simulink model "NewOrbitSimulation"  (R2015a)
settings: Solver=ode45  StartTime=0.0  StopTime=1000  FixedStep=.1  RelTol=1e-9
InitFcn:
  | PlanetSelect;
StopFcn:
  | TotalDeltaV
values from neighbouring files (symbols this model uses):
  Aero_On = 1    [PlanetSelect.m]
  AtmoData = 0    [PlanetSelect.m]
  Cd = 2    [PlanetSelect.m]
  Cl = 2    [PlanetSelect.m]
  Coasting_Parameter = 306.412    [PlanetSelect.m]
  Constant_Drag_On = 1    [PlanetSelect.m]
  Constant_Lift_On = 1    [PlanetSelect.m]
  CraftInitialP = [Px;Py]    [PlanetSelect.m]
  CraftInitialV = [Vx;Vy]    [PlanetSelect.m]
  Drag_On = 1    [PlanetSelect.m]
  g0 = 9.80665    [PlanetSelect.m]
  LastStage = size(ThrustMassData,1)    [PlanetSelect.m]
  Lift_On = 0    [PlanetSelect.m]
  PitchOverAlt = 1000    [PlanetSelect.m]
  PitchOverAngle = 7.5    [PlanetSelect.m]
  PitchSwitch = .5    (= 0.5)    [PlanetSelect.m]
  RefSurfArea = 10.8    [PlanetSelect.m]
  TargetOrbit = 100000-GndAlt_planet    [PlanetSelect.m]
  Throttle = 1.5*g0*ThrustMassData(1,1)/(1000*ThrustMassData(1,3))    [PlanetSelect.m]
  ThrustEnable = 1    [PlanetSelect.m]
undefined symbols (not defined in the file or in its folder): AtmoAlt_planet, DragData, GM_planet, GndAlt_planet, Omega_planet, R_planet
libraries: simulink_extras x6, dspmathops x5, simulink x3, vrlib x2
settings Model: PauseTimes=122  SnapshotInterval=1  Creator=raulm_000  LastModifiedBy=raulm_000
settings DataIOCC: ExternalInput=[Throttle,SSIGN]  LimitDataPoints=off  SaveFinalState=on

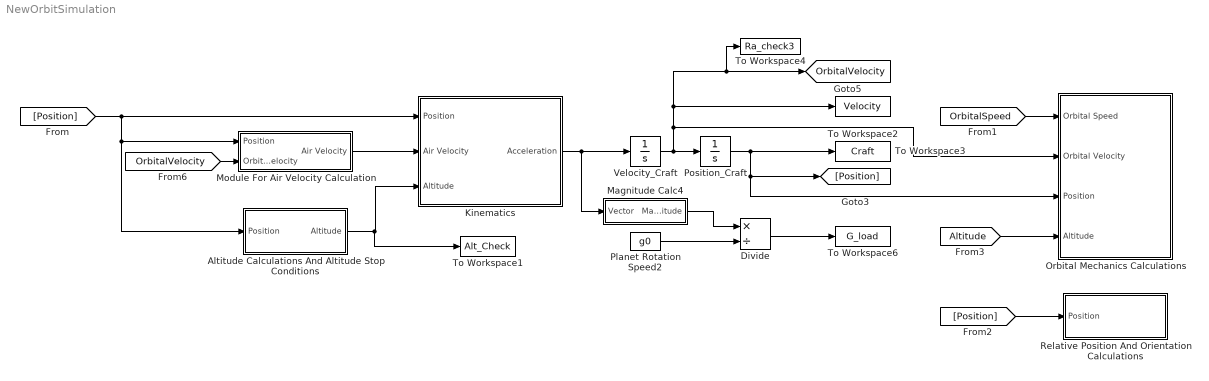
== system NewOrbitSimulation ==
  Altitude Calculations And Altitude Stop Conditions : Subsystem
  Divide : Product  Inputs=*/
  Kinematics : Subsystem
  Magnitude Calc4 : Subsystem
  Module For Air Velocity Calculation : Subsystem
  Orbital Mechanics Calculations : Subsystem
  Planet Rotation Speed2 : Constant  Value=g0
  Position_Craft : Integrator  InitialCondition=CraftInitialP
  Relative Position And Orientation Calculations : Subsystem
  To Workspace1 : ToWorkspace  VariableName=Alt_Check  SampleTime=-1
      settings: MaxDataPoints=1
  To Workspace2 : ToWorkspace  VariableName=Velocity  SampleTime=-1
  To Workspace3 : ToWorkspace  VariableName=Craft  SampleTime=-1
  To Workspace4 : ToWorkspace  VariableName=Ra_check3  SampleTime=-1
      settings: MaxDataPoints=1
  To Workspace6 : ToWorkspace  VariableName=G_load  SampleTime=-1
  Velocity_Craft : Integrator  InitialCondition=CraftInitialV-[.1;0]
  tag scope: OrbitalVelocity=global
  wires:
  Velocity_Craft/1 -> Position_Craft/1, To Workspace4/1, [OrbitalVelocity], To Workspace2/1, Orbital Mechanics Calculations/2(Orbital Velocity)
  Kinematics/1("Acceleration ") -> Velocity_Craft/1, Magnitude Calc4/1(Vector)
  Magnitude Calc4/1("Magnitude ") -> Divide/1
  Planet Rotation Speed2/1 -> Divide/2
  Divide/1 -> To Workspace6/1
  [OrbitalSpeed] -> Orbital Mechanics Calculations/1(Orbital Speed)
  [Altitude] -> Orbital Mechanics Calculations/4(Altitude)
  Position_Craft/1 -> Orbital Mechanics Calculations/3(Position), [Position], To Workspace3/1
  Module For Air Velocity Calculation/1(Air Velocity) -> Kinematics/2(Air Velocity)
  [Position] -> Module For Air Velocity Calculation/1(Position), Altitude Calculations And Altitude Stop Conditions/1(Position), Kinematics/1(Position)
  Altitude Calculations And Altitude Stop Conditions/1(Altitude) -> To Workspace1/1, Kinematics/3("Altitude ")
  [OrbitalVelocity] -> Module For Air Velocity Calculation/2(Orbital Velocity)
  [Position] -> Relative Position And Orientation Calculations/1(Position)

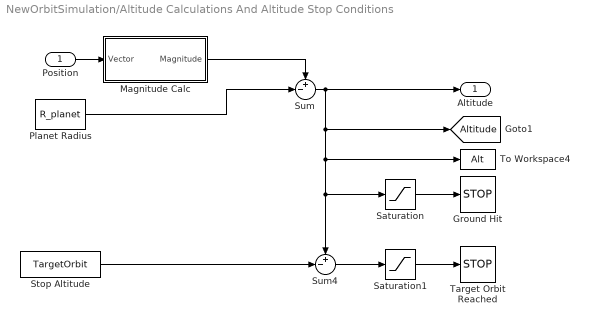
== system NewOrbitSimulation/Altitude Calculations And Altitude Stop Conditions ==
  Position : Inport
  " Target Orbit Reached" : Stop
  Ground Hit : Stop
  Magnitude Calc : Subsystem
  "Planet Radius " : Constant  Value=R_planet
  Saturation : Saturate  UpperLimit=0
  Saturation1 : Saturate  UpperLimit=1  LowerLimit=0
  Stop Altitude : Constant  Value=TargetOrbit
  Sum : Sum  Inputs=+-|
  Sum4 : Sum  Inputs=+-|
  To Workspace4 : ToWorkspace  VariableName=Alt  SampleTime=-1
  Altitude : Outport
  tag scope: Altitude=global
  wires:
  Magnitude Calc/1("Magnitude ") -> Sum/1
  "Planet Radius "/1 -> Sum/2
  Sum/1 -> Sum4/1, Saturation/1, To Workspace4/1, [Altitude], Altitude/1
  Saturation/1 -> Ground Hit/1
  Stop Altitude/1 -> Sum4/2
  Sum4/1 -> Saturation1/1
  Saturation1/1 -> " Target Orbit Reached"/1
  Position/1 -> Magnitude Calc/1(Vector)

== system NewOrbitSimulation/Kinematics ==
  Position : Inport
  Air Velocity : Inport  Port=2
  "Altitude " : Inport  Port=3
  Aerodynamics : Subsystem
  Gravitational Acceleration : Subsystem
  Sum3 : Sum  Inputs=+++
  Thrust : Subsystem
  "Acceleration " : Outport
  wires:
  Position/1 -> Thrust/2(Position), Gravitational Acceleration/1(Position)
  Air Velocity/1 -> Thrust/3(AirVelocity), Aerodynamics/1(Air Velocity)
  "Altitude "/1 -> Thrust/1(Altitude), Aerodynamics/2("Altitude ")
  Aerodynamics/1("Aeroaccel ") -> Sum3/2
  Gravitational Acceleration/1("Gavity ") -> Sum3/1
  Sum3/1 -> "Acceleration "/1
  Thrust/1("ThrustAccel ") -> Sum3/3

== system NewOrbitSimulation/Magnitude Calc4 ==
  Vector : Inport
  Add : Sum
  Demux : Demux  Outputs=2
  Math Function : Math  Operator=square  SaturateOnIntegerOverflow=on
  Math Function1 : Math  Operator=square  SaturateOnIntegerOverflow=on
  Sqrt : Sqrt  SaturateOnIntegerOverflow=on
  "Magnitude " : Outport
  wires:
  Demux/1 -> Math Function1/1
  Demux/2 -> Math Function/1
  Math Function/1 -> Add/2
  Add/1 -> Sqrt/1
  Vector/1 -> Demux/1
  Math Function1/1 -> Add/1
  Sqrt/1 -> "Magnitude "/1

== system NewOrbitSimulation/Module For Air Velocity Calculation ==
  Position : Inport
  Orbital Velocity : Inport  Port=2
  Cross Product1 : vrlib/Utilities/Cross Product
  Magnitude Calc1 : Subsystem
  Magnitude Calc3 : Subsystem
  Mux : Mux  Inputs=2
  Planet Rotation Speed1 : Constant  Value=0
  Sum2 : Sum  Inputs=|-+
  Air Velocity : Outport
  tag scope: OrbitalSpeed=global
  wires:
  [Planet_Ang_Vec] -> Cross Product1/1
  Cross Product1/1 -> Magnitude Calc3/1(3-in)
  Mux/1 -> Cross Product1/2
  Planet Rotation Speed1/1 -> Mux/2
  Magnitude Calc3/1("2-out ") -> Sum2/1
  Magnitude Calc1/1("Magnitude ") -> [OrbitalSpeed]
  Orbital Velocity/1 -> Sum2/2, Magnitude Calc1/1(Vector)
  Position/1 -> Mux/1
  Sum2/1 -> Air Velocity/1

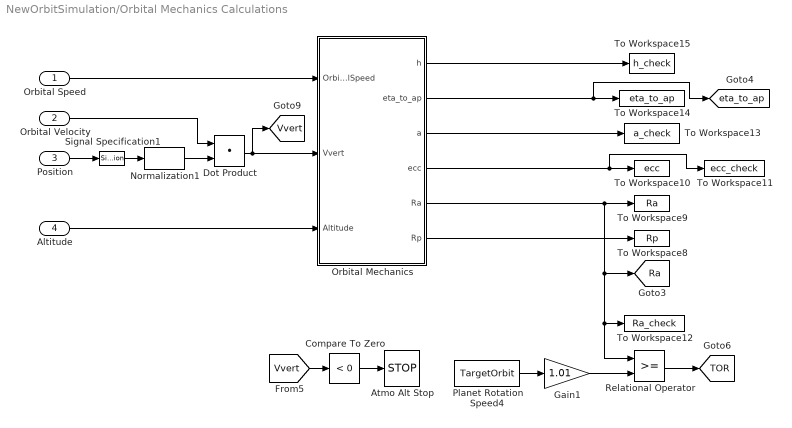
== system NewOrbitSimulation/Orbital Mechanics Calculations ==
  Orbital Speed : Inport
  Orbital Velocity : Inport  Port=2
  Position : Inport  Port=3
  Altitude : Inport  Port=4
  Atmo Alt Stop : Stop
  Compare To Zero : simulink/Logic and Bit Operations/Compare To Zero  relop=<  OutDataTypeStr=boolean
  Dot Product : DotProduct  InputSameDT=on  OutDataTypeStr=Inherit: Inherit via internal rule
  Gain1 : Gain  Gain=1.01
  Normalization1 : dspmathops/Normalization  NormType=2-norm  Bias=1e-10  NormOver=Specified dimension  ColComp=off  Dimension=1  outputMin=[]  outputMax=[]  accumDataTypeStr=Inherit: Same as product output  accumLastDataTypeStr=Inherit: Same as product output  roundingMode=Floor  overflowMode=off
  Orbital Mechanics : MATLAB Function  TreatAsAtomicUnit=on
  Planet Rotation Speed4 : Constant  Value=TargetOrbit
  Relational Operator : RelationalOperator  OutDataTypeStr=boolean
  Signal Specification1 : SignalSpecification  Dimensions=2
  To Workspace10 : ToWorkspace  VariableName=ecc  SampleTime=-1
  To Workspace11 : ToWorkspace  VariableName=ecc_check  SampleTime=-1
      settings: MaxDataPoints=1
  To Workspace12 : ToWorkspace  VariableName=Ra_check  SampleTime=-1
      settings: MaxDataPoints=1
  To Workspace13 : ToWorkspace  VariableName=a_check  SampleTime=-1
      settings: MaxDataPoints=1
  To Workspace14 : ToWorkspace  VariableName=eta_to_ap  SampleTime=-1
  To Workspace15 : ToWorkspace  VariableName=h_check  SampleTime=-1
      settings: MaxDataPoints=1
  To Workspace8 : ToWorkspace  VariableName=Rp  SampleTime=-1
  To Workspace9 : ToWorkspace  VariableName=Ra  SampleTime=-1
  tag scope: Ra=global, TOR=global, Vvert=global, eta_to_ap=global
  wires:
  Orbital Mechanics/5(Ra) -> Relational Operator/1, To Workspace12/1, [Ra], To Workspace9/1
  Orbital Mechanics/6(Rp) -> To Workspace8/1
  Orbital Mechanics/4(ecc) -> To Workspace10/1, To Workspace11/1
  Planet Rotation Speed4/1 -> Gain1/1
  Relational Operator/1 -> [TOR]
  Orbital Mechanics/3(a) -> To Workspace13/1
  Orbital Mechanics/2(eta_to_ap) -> [eta_to_ap], To Workspace14/1
  Orbital Mechanics/1(h) -> To Workspace15/1
  Orbital Velocity/1 -> Dot Product/1
  Dot Product/1 -> Orbital Mechanics/2(Vvert), [Vvert]
  Gain1/1 -> Relational Operator/2
  [Vvert] -> Compare To Zero/1
  Compare To Zero/1 -> Atmo Alt Stop/1
  Signal Specification1/1 -> Normalization1/1
  Orbital Speed/1 -> Orbital Mechanics/1(OrbitalSpeed)
  Position/1 -> Signal Specification1/1
  Normalization1/1 -> Dot Product/2
  Altitude/1 -> Orbital Mechanics/3(Altitude)

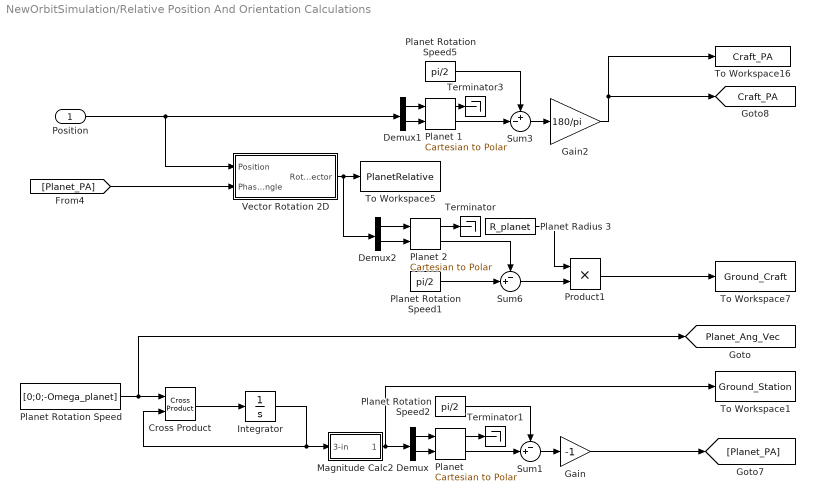
== system NewOrbitSimulation/Relative Position And Orientation Calculations ==
  Position : Inport
  Cross Product : vrlib/Utilities/Cross Product
  Demux : Demux  Outputs=2
  Demux1 : Demux  Outputs=2
  Demux2 : Demux  Outputs=2
  Gain : Gain  Gain=-1
  Gain2 : Gain  Gain=180/pi
  Integrator : Integrator  InitialCondition=[0;R_planet;0]
  Magnitude Calc2 : Subsystem
  "Planet " : simulink_extras/Transformations/Cartesian to Polar
  Planet 1 : simulink_extras/Transformations/Cartesian to Polar
  Planet 2 : simulink_extras/Transformations/Cartesian to Polar
  Planet Radius 3 : Constant  Value=R_planet
  Planet Rotation Speed : Constant  Value=[0;0;-Omega_planet]
  Planet Rotation Speed1 : Constant  Value=pi/2
  Planet Rotation Speed2 : Constant  Value=pi/2
  Planet Rotation Speed5 : Constant  Value=pi/2
  Product1 : Product
  Sum1 : Sum  Inputs=-+|
  Sum3 : Sum  Inputs=+-|
  Sum6 : Sum  Inputs=-+|
  Terminator : Terminator
  Terminator1 : Terminator
  Terminator3 : Terminator
  To Workspace1 : ToWorkspace  VariableName=Ground_Station  SampleTime=-1
  To Workspace16 : ToWorkspace  VariableName=Craft_PA  SampleTime=-1
  To Workspace5 : ToWorkspace  VariableName=PlanetRelative  SampleTime=-1
  To Workspace7 : ToWorkspace  VariableName=Ground_Craft  SampleTime=-1
  Vector Rotation 2D : Subsystem
  tag scope: Craft_PA=global, Planet_Ang_Vec=global
  wires:
  Planet Rotation Speed/1 -> [Planet_Ang_Vec], Cross Product/1
  Integrator/1 -> Cross Product/2, Magnitude Calc2/1(3-in)
  Cross Product/1 -> Integrator/1
  Magnitude Calc2/1("2-out ") -> To Workspace1/1, Demux/1
  Demux/1 -> "Planet "/1
  Demux/2 -> "Planet "/2
  Vector Rotation 2D/1("Rotated Vector ") -> Demux2/1, To Workspace5/1
  "Planet "/2 -> Sum1/2
  Planet Rotation Speed2/1 -> Sum1/1
  Sum1/1 -> Gain/1
  Planet 2/2 -> Sum6/1
  Planet Radius 3/1 -> Product1/1
  Product1/1 -> To Workspace7/1
  Planet Rotation Speed1/1 -> Sum6/2
  Sum6/1 -> Product1/2
  Demux2/1 -> Planet 2/1
  Demux2/2 -> Planet 2/2
  Planet 2/1 -> Terminator/1
  "Planet "/1 -> Terminator1/1
  Gain/1 -> [Planet_PA]
  [Planet_PA] -> Vector Rotation 2D/2(Phase Angle)
  Demux1/1 -> Planet 1/1
  Demux1/2 -> Planet 1/2
  Planet 1/2 -> Sum3/2
  Planet Rotation Speed5/1 -> Sum3/1
  Planet 1/1 -> Terminator3/1
  Sum3/1 -> Gain2/1
  Gain2/1 -> To Workspace16/1, [Craft_PA]
  Position/1 -> Vector Rotation 2D/1(Position), Demux1/1

== system NewOrbitSimulation/Altitude Calculations And Altitude Stop Conditions/Magnitude Calc ==
  Vector : Inport
  Add : Sum
  Demux : Demux  Outputs=2
  Math Function : Math  Operator=square  SaturateOnIntegerOverflow=on
  Math Function1 : Math  Operator=square  SaturateOnIntegerOverflow=on
  Sqrt : Sqrt  SaturateOnIntegerOverflow=on
  "Magnitude " : Outport
  wires:
  Demux/1 -> Math Function1/1
  Demux/2 -> Math Function/1
  Math Function/1 -> Add/2
  Add/1 -> Sqrt/1
  Vector/1 -> Demux/1
  Math Function1/1 -> Add/1
  Sqrt/1 -> "Magnitude "/1

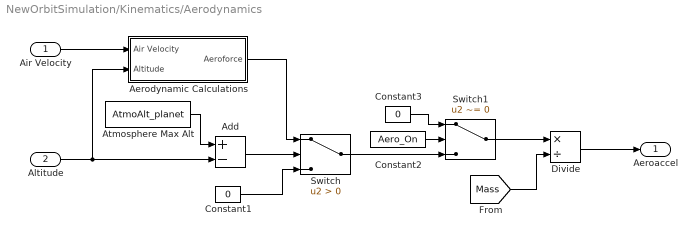
== system NewOrbitSimulation/Kinematics/Aerodynamics ==
  Air Velocity : Inport
  "Altitude " : Inport  Port=2
  Add : Sum  Inputs=+-
  Aerodynamic Calculations : Subsystem
  Atmosphere Max Alt : Constant  Value=AtmoAlt_planet
  Constant1 : Constant  Value=0
  Constant2 : Constant  Value=Aero_On
  Constant3 : Constant  Value=0
  Divide : Product  Inputs=*/
  Switch : Switch  Criteria=u2 > Threshold
  Switch1 : Switch  Criteria=u2 ~= 0
  "Aeroaccel " : Outport
  wires:
  "Altitude "/1 -> Aerodynamic Calculations/2(Altitude), Add/2
  Atmosphere Max Alt/1 -> Add/1
  Add/1 -> Switch/2
  Constant1/1 -> Switch/3
  Divide/1 -> "Aeroaccel "/1
  [Mass] -> Divide/2
  Air Velocity/1 -> Aerodynamic Calculations/1(Air Velocity)
  Aerodynamic Calculations/1("Aeroforce ") -> Switch/1
  Switch1/1 -> Divide/1
  Switch/1 -> Switch1/3
  Constant2/1 -> Switch1/2
  Constant3/1 -> Switch1/1

== system NewOrbitSimulation/Kinematics/Gravitational Acceleration ==
  Position : Inport
  Divide : Product  Inputs=*/
  Gain : Gain  Gain=-1
  Magnitude Calc : Subsystem
  Math Function : Math  Operator=square  SaturateOnIntegerOverflow=on
  Normalization : dspmathops/Normalization  NormType=2-norm  Bias=1e-10  NormOver=Specified dimension  ColComp=off  Dimension=1  outputDataTypeStr=Inherit: Same as product output  outputLastDataTypeStr=Inherit: Same as product output  outputMin=[]  outputMax=[]  accumDataTypeStr=Inherit: Same as product output  accumLastDataTypeStr=Inherit: Same as product output  roundingMode=Floor  overflowMode=off
  Planet GM : Constant  Value=GM_planet
  Product : Product
  "Gavity " : Outport
  wires:
  Position/1 -> Normalization/1, Magnitude Calc/1(Vector)
  Magnitude Calc/1("Magnitude ") -> Math Function/1
  Planet GM/1 -> Divide/1
  Math Function/1 -> Divide/2
  Product/1 -> "Gavity "/1
  Gain/1 -> Product/2
  Divide/1 -> Product/1
  Normalization/1 -> Gain/1

== system NewOrbitSimulation/Kinematics/Thrust ==
  Altitude : Inport
  Position : Inport  Port=2
  AirVelocity : Inport  Port=3
  Divide : Product  Inputs=*/
  Mass and fuel consumption : Subsystem
  Pitch Calculation : Subsystem
  Product1 : Product
  To Workspace1 : ToWorkspace  VariableName=Mass  SampleTime=-1
  "ThrustAccel " : Outport
  tag scope: Mass=global
  wires:
  Product1/1 -> Divide/1
  Mass and fuel consumption/1("Mass ") -> To Workspace1/1, [Mass]
  [Mass] -> Divide/2
  Mass and fuel consumption/2("Thrust ") -> Product1/1
  Position/1 -> Pitch Calculation/2(Position)
  Pitch Calculation/1(Thrust Vector) -> Product1/2
  Altitude/1 -> Pitch Calculation/1(Altitude)
  AirVelocity/1 -> Pitch Calculation/3(AirVelocity)
  Divide/1 -> "ThrustAccel "/1

== system NewOrbitSimulation/Module For Air Velocity Calculation/Magnitude Calc1 ==
  Vector : Inport
  Add : Sum
  Demux : Demux  Outputs=2
  Math Function : Math  Operator=square  SaturateOnIntegerOverflow=on
  Math Function1 : Math  Operator=square  SaturateOnIntegerOverflow=on
  Sqrt : Sqrt  SaturateOnIntegerOverflow=on
  "Magnitude " : Outport
  wires:
  Demux/1 -> Math Function1/1
  Demux/2 -> Math Function/1
  Math Function/1 -> Add/2
  Add/1 -> Sqrt/1
  Vector/1 -> Demux/1
  Math Function1/1 -> Add/1
  Sqrt/1 -> "Magnitude "/1

== system NewOrbitSimulation/Module For Air Velocity Calculation/Magnitude Calc3 ==
  3-in : Inport
  Demux4 : Demux  Outputs=3
  Mux2 : Mux  Inputs=2
  Terminator3 : Terminator
  "2-out " : Outport
  wires:
  3-in/1 -> Demux4/1
  Demux4/3 -> Terminator3/1
  Demux4/1 -> Mux2/1
  Demux4/2 -> Mux2/2
  Mux2/1 -> "2-out "/1

== system NewOrbitSimulation/Relative Position And Orientation Calculations/Magnitude Calc2 ==
  3-in : Inport
  Demux4 : Demux  Outputs=3
  Mux2 : Mux  Inputs=2
  Terminator3 : Terminator
  "2-out " : Outport
  wires:
  3-in/1 -> Demux4/1
  Demux4/3 -> Terminator3/1
  Demux4/1 -> Mux2/1
  Demux4/2 -> Mux2/2
  Mux2/1 -> "2-out "/1

== system NewOrbitSimulation/Relative Position And Orientation Calculations/Vector Rotation 2D ==
  Position : Inport
  Phase Angle : Inport  Port=2
  Add : Sum  Inputs=+-
  Add1 : Sum
  Demux : Demux  Outputs=2
  Mux : Mux  Inputs=2
  Product{,1..3} (4 alike) : Product
  Trigonometric Function : Trigonometry
  Trigonometric Function1 : Trigonometry  Operator=cos
  "Rotated Vector " : Outport
  wires:
  Mux/1 -> "Rotated Vector "/1
  Phase Angle/1 -> Trigonometric Function/1, Trigonometric Function1/1
  Position/1 -> Demux/1
  Trigonometric Function1/1 -> Product3/2, Product/2
  Demux/1 -> Product2/2, Product/1
  Product/1 -> Add/1
  Demux/2 -> Product3/1, Product1/1
  Trigonometric Function/1 -> Product2/1, Product1/2
  Product1/1 -> Add/2
  Product2/1 -> Add1/1
  Product3/1 -> Add1/2
  Add1/1 -> Mux/2
  Add/1 -> Mux/1

== system NewOrbitSimulation/Kinematics/Aerodynamics/Aerodynamic Calculations ==
  Air Velocity : Inport
  Altitude : Inport  Port=2
  Cl and Cd Calculation : Subsystem
  Magnitude Calc1 : Subsystem
  Product : Product  Inputs=3
  Referance Surface Area : Constant  Value=RefSurfArea
  "Aeroforce " : Outport
  wires:
  Air Velocity/1 -> Cl and Cd Calculation/1(Air Velocity), Magnitude Calc1/1(Air Velocity)
  Altitude/1 -> Cl and Cd Calculation/2("Altitude "), Magnitude Calc1/2("Altitude ")
  Product/1 -> "Aeroforce "/1
  Magnitude Calc1/1("Dynamic Pressure ") -> Product/1
  Cl and Cd Calculation/1(Cl + Cd) -> Product/2
  Referance Surface Area/1 -> Product/3

== system NewOrbitSimulation/Kinematics/Gravitational Acceleration/Magnitude Calc ==
  Vector : Inport
  Add : Sum
  Demux : Demux  Outputs=2
  Math Function : Math  Operator=square  SaturateOnIntegerOverflow=on
  Math Function1 : Math  Operator=square  SaturateOnIntegerOverflow=on
  Sqrt : Sqrt  SaturateOnIntegerOverflow=on
  "Magnitude " : Outport
  wires:
  Demux/1 -> Math Function1/1
  Demux/2 -> Math Function/1
  Math Function/1 -> Add/2
  Add/1 -> Sqrt/1
  Vector/1 -> Demux/1
  Math Function1/1 -> Add/1
  Sqrt/1 -> "Magnitude "/1

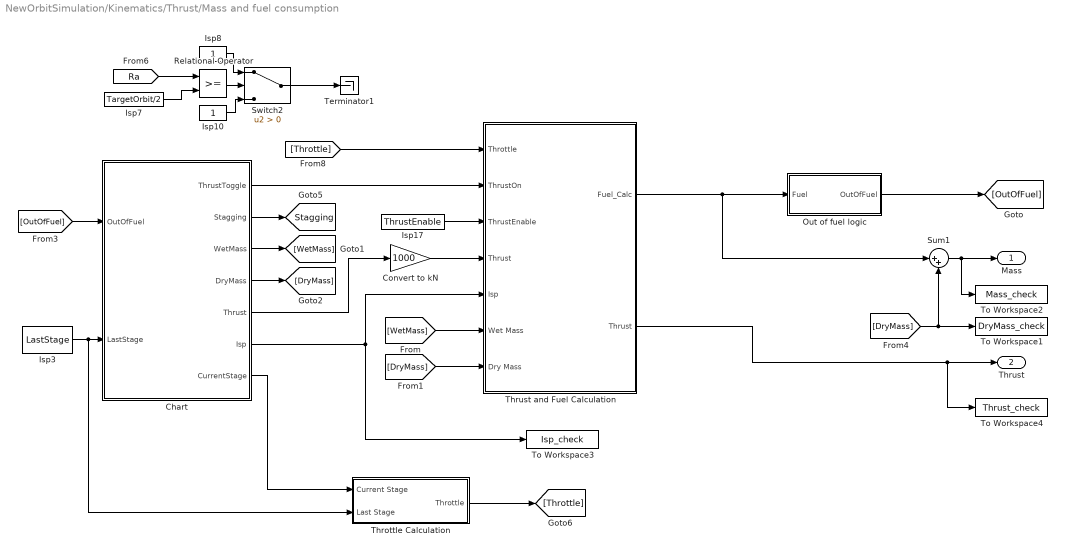
== system NewOrbitSimulation/Kinematics/Thrust/Mass and fuel consumption ==
  Chart : Stateflow chart  TreatAsAtomicUnit=on
  Convert to kN : Gain  Gain=1000
  Isp10 : Constant
  Isp17 : Constant  Value=ThrustEnable
  Isp3 : Constant  Value=LastStage
  Isp7 : Constant  Value=TargetOrbit/2
  Isp8 : Constant
  Out of fuel logic : Subsystem
  Relational Operator : RelationalOperator  OutDataTypeStr=boolean
  Sum1 : Sum  Inputs=|++
  Switch2 : Switch  Criteria=u2 > Threshold
  Terminator1 : Terminator
  Throttle Calculation : Subsystem
  Thrust and Fuel Calculation : Subsystem
  To Workspace1 : ToWorkspace  VariableName=DryMass_check  SampleTime=-1
      settings: MaxDataPoints=1
  To Workspace2 : ToWorkspace  VariableName=Mass_check  SampleTime=-1
      settings: MaxDataPoints=1
  To Workspace3 : ToWorkspace  VariableName=Isp_check  SampleTime=-1
      settings: MaxDataPoints=1
  To Workspace4 : ToWorkspace  VariableName=Thrust_check  SampleTime=-1
      settings: MaxDataPoints=1
  "Mass " : Outport
  "Thrust " : Outport  Port=2
  tag scope: Stagging=global
  wires:
  Sum1/1 -> To Workspace2/1, "Mass "/1
  [DryMass] -> Sum1/2, To Workspace1/1
  [OutOfFuel] -> Chart/1(OutOfFuel)
  Isp3/1 -> Throttle Calculation/2(Last Stage), Chart/2(LastStage)
  Chart/2(Stagging) -> [Stagging]
  Chart/3(WetMass) -> [WetMass]
  Chart/4(DryMass) -> [DryMass]
  Chart/5(Thrust) -> Convert to kN/1
  Chart/6(Isp) -> To Workspace3/1, Thrust and Fuel Calculation/5(Isp)
  Isp7/1 -> Relational Operator/2
  [Ra] -> Relational Operator/1
  Relational Operator/1 -> Switch2/2
  Isp10/1 -> Switch2/3
  Isp8/1 -> Switch2/1
  Chart/1(ThrustToggle) -> Thrust and Fuel Calculation/2(ThrustOn)
  Switch2/1 -> Terminator1/1
  Convert to kN/1 -> Thrust and Fuel Calculation/4(Thrust)
  [Throttle] -> Thrust and Fuel Calculation/1(Throttle)
  Isp17/1 -> Thrust and Fuel Calculation/3(ThrustEnable)
  Thrust and Fuel Calculation/2("Thrust ") -> To Workspace4/1, "Thrust "/1
  [DryMass] -> Thrust and Fuel Calculation/7(Dry Mass)
  [WetMass] -> Thrust and Fuel Calculation/6(Wet Mass)
  Throttle Calculation/1(Throttle) -> [Throttle]
  Chart/7(CurrentStage) -> Throttle Calculation/1(Current Stage)
  Thrust and Fuel Calculation/1(Fuel_Calc) -> Sum1/1, Out of fuel logic/1(Fuel)
  Out of fuel logic/1(OutOfFuel) -> [OutOfFuel]

== system NewOrbitSimulation/Kinematics/Thrust/Pitch Calculation ==
  Altitude : Inport  PortDimensions=1
  Position : Inport  Port=2
  AirVelocity : Inport  Port=3
  Constant : Constant  Value=PitchOverAlt
  Gravity Turn Pitch Calculation : Subsystem
  Relational Operator : RelationalOperator  OutDataTypeStr=boolean
  Subsystem : Subsystem
  Switch1 : Switch  Criteria=u2 ~= 0  Threshold=PitchOverAlt
  Thrust Vector Scope : Scope
  Thrust Vector : Outport
  wires:
  Relational Operator/1 -> Switch1/2
  Constant/1 -> Relational Operator/1
  Altitude/1 -> Subsystem/2(Altitude), Relational Operator/2
  Switch1/1 -> Thrust Vector/1, Thrust Vector Scope/1
  Position/1 -> Subsystem/1(Position)
  Subsystem/1(Up Vector) -> Switch1/1
  AirVelocity/1 -> Gravity Turn Pitch Calculation/1(Air Velocity)
  Gravity Turn Pitch Calculation/1(Thrust Vec) -> Switch1/3

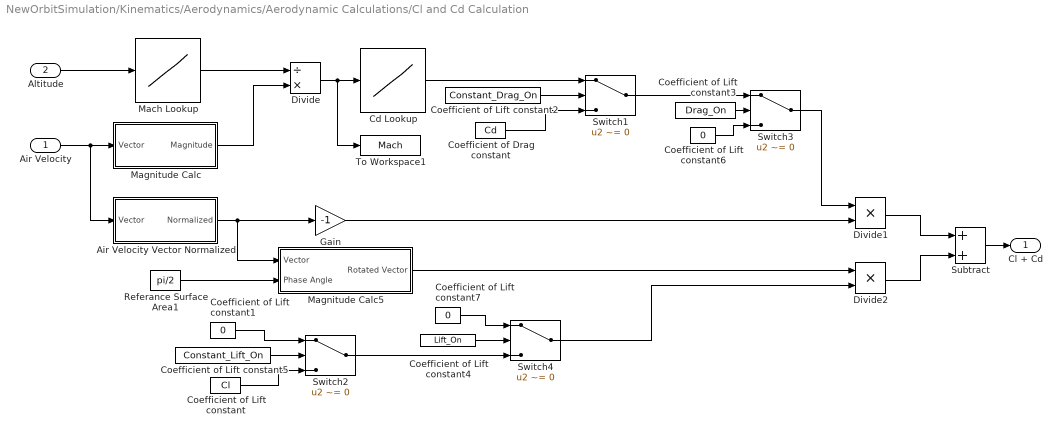
== system NewOrbitSimulation/Kinematics/Aerodynamics/Aerodynamic Calculations/Cl and Cd Calculation ==
  Air Velocity : Inport
  "Altitude " : Inport  Port=2
  Air Velocity Vector Normalized : Subsystem
  Cd Lookup : Lookup_n-D  NumberOfTableDimensions=1  BreakpointsForDimension1=DragData(:,1)  Table=DragData(:,2)  InternalRulePriority=Speed  RndMeth=Simplest  InputSameDT=on
  Coefficient of Drag constant : Constant  Value=Cd
  Coefficient of Lift constant : Constant  Value=Cl
  Coefficient of Lift constant1 : Constant  Value=0
  Coefficient of Lift constant2 : Constant  Value=Constant_Drag_On
  Coefficient of Lift constant3 : Constant  Value=Drag_On
  Coefficient of Lift constant4 : Constant  Value=Lift_On
  Coefficient of Lift constant5 : Constant  Value=Constant_Lift_On
  Coefficient of Lift constant6 : Constant  Value=0
  Coefficient of Lift constant7 : Constant  Value=0
  Divide : Product  Inputs=/*
  Divide1 : Product  Inputs=**
  Divide2 : Product  Inputs=**
  Gain : Gain  Gain=-1
  Mach Lookup : Lookup_n-D  NumberOfTableDimensions=1  BreakpointsForDimension1=AtmoData(:,1)  Table=AtmoData(:,4)  InternalRulePriority=Speed  RndMeth=Simplest  InputSameDT=on
  Magnitude Calc : Subsystem
  Magnitude Calc5 : Subsystem
  Referance Surface Area1 : Constant  Value=pi/2
  Subtract : Sum
  Switch{1..4} (4 alike) : Switch  Criteria=u2 ~= 0
  To Workspace1 : ToWorkspace  VariableName=Mach  SampleTime=-1
  Cl + Cd : Outport
  wires:
  "Altitude "/1 -> Mach Lookup/1
  Air Velocity/1 -> Air Velocity Vector Normalized/1(Vector), Magnitude Calc/1(Vector)
  Magnitude Calc/1("Magnitude ") -> Divide/2
  Mach Lookup/1 -> Divide/1
  Divide/1 -> To Workspace1/1, Cd Lookup/1
  Air Velocity Vector Normalized/1("Normalized ") -> Magnitude Calc5/1(Vector), Gain/1
  Gain/1 -> Divide1/2
  Divide1/1 -> Subtract/1
  Referance Surface Area1/1 -> Magnitude Calc5/2(Phase Angle)
  Magnitude Calc5/1("Rotated Vector ") -> Divide2/1
  Coefficient of Lift constant2/1 -> Switch1/2
  Switch3/1 -> Divide1/1
  Subtract/1 -> Cl + Cd/1
  Coefficient of Drag constant/1 -> Switch1/3
  Cd Lookup/1 -> Switch1/1
  Coefficient of Lift constant5/1 -> Switch2/2
  Coefficient of Lift constant1/1 -> Switch2/1
  Coefficient of Lift constant/1 -> Switch2/3
  Coefficient of Lift constant3/1 -> Switch3/2
  Coefficient of Lift constant6/1 -> Switch3/3
  Switch1/1 -> Switch3/1
  Coefficient of Lift constant4/1 -> Switch4/2
  Switch2/1 -> Switch4/3
  Coefficient of Lift constant7/1 -> Switch4/1
  Switch4/1 -> Divide2/2
  Divide2/1 -> Subtract/2

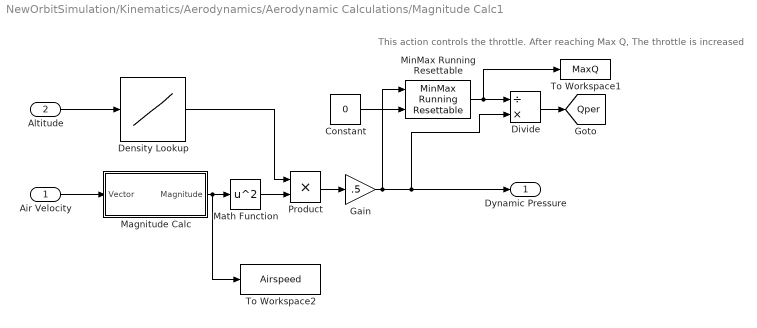
== system NewOrbitSimulation/Kinematics/Aerodynamics/Aerodynamic Calculations/Magnitude Calc1 ==
  note: This action controls the throttle. After reaching Max Q, The throttle is increased
  Air Velocity : Inport
  "Altitude " : Inport  Port=2
  Constant : Constant  Value=0
  Density Lookup : Lookup_n-D  NumberOfTableDimensions=1  BreakpointsForDimension1=AtmoData(:,1)  Table=AtmoData(:,3)  InternalRulePriority=Speed  RndMeth=Simplest  InputSameDT=on
  Divide : Product  Inputs=/*
  Gain : Gain  Gain=.5
  Magnitude Calc : Subsystem
  Math Function : Math  Operator=square  SaturateOnIntegerOverflow=on
  MinMax Running Resettable : simulink/Math Operations/MinMax Running Resettable  Function=max  vinit=0.0
  Product : Product
  To Workspace1 : ToWorkspace  VariableName=MaxQ  SampleTime=-1
      settings: MaxDataPoints=1
  To Workspace2 : ToWorkspace  VariableName=Airspeed  SampleTime=-1
  "Dynamic Pressure " : Outport
  tag scope: Qper=global
  wires:
  "Altitude "/1 -> Density Lookup/1
  Magnitude Calc/1("Magnitude ") -> To Workspace2/1, Math Function/1
  Air Velocity/1 -> Magnitude Calc/1(Vector)
  Math Function/1 -> Product/2
  Product/1 -> Gain/1
  Density Lookup/1 -> Product/1
  MinMax Running Resettable/1 -> To Workspace1/1, Divide/1
  Constant/1 -> MinMax Running Resettable/2
  Gain/1 -> MinMax Running Resettable/1, Divide/2, "Dynamic Pressure "/1
  Divide/1 -> [Qper]

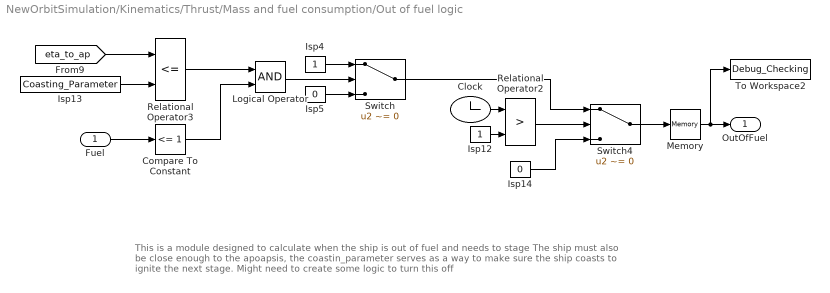
== system NewOrbitSimulation/Kinematics/Thrust/Mass and fuel consumption/Out of fuel logic ==
  note: This is a module designed to calculate when the ship is out of fuel and needs to stage
      |
      | The ship must also be close enough to the apoapsis, the coastin_parameter serves as a
      | way to make sure the ship coasts to ignite the next stage. Might need to create some logic to turn this off
  Fuel : Inport
  Clock : Clock
  Compare To Constant : simulink/Logic and Bit Operations/Compare To Constant  relop=<=  const=1  OutDataTypeStr=boolean
  Isp12 : Constant
  Isp13 : Constant  Value=Coasting_Parameter
  Isp14 : Constant  Value=0
  Isp4 : Constant
  Isp5 : Constant  Value=0
  Logical Operator : Logic  AllPortsSameDT=off  OutDataTypeStr=boolean
  Memory : Memory
  Relational Operator2 : RelationalOperator  Operator=>  OutDataTypeStr=boolean
  Relational Operator3 : RelationalOperator  Operator=<=  OutDataTypeStr=boolean
  Switch : Switch  Criteria=u2 ~= 0
  Switch4 : Switch  Criteria=u2 ~= 0
  To Workspace2 : ToWorkspace  VariableName=Debug_Checking  SampleTime=-1
      settings: MaxDataPoints=1
  OutOfFuel : Outport
  wires:
  Isp4/1 -> Switch/1
  Isp5/1 -> Switch/3
  [eta_to_ap] -> Relational Operator3/1
  Isp13/1 -> Relational Operator3/2
  Relational Operator3/1 -> Logical Operator/1
  Clock/1 -> Relational Operator2/1
  Isp12/1 -> Relational Operator2/2
  Relational Operator2/1 -> Switch4/2
  Switch/1 -> Switch4/1
  Isp14/1 -> Switch4/3
  Switch4/1 -> Memory/1
  Memory/1 -> To Workspace2/1, OutOfFuel/1
  Compare To Constant/1 -> Logical Operator/2
  Logical Operator/1 -> Switch/2
  Fuel/1 -> Compare To Constant/1

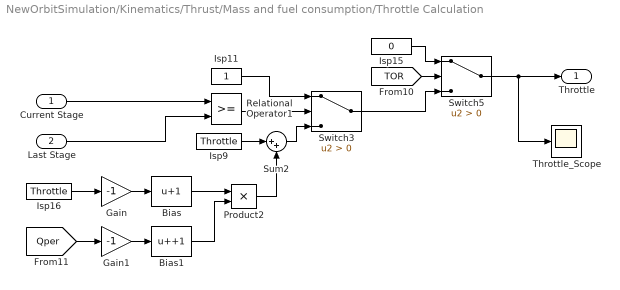
== system NewOrbitSimulation/Kinematics/Thrust/Mass and fuel consumption/Throttle Calculation ==
  Current Stage : Inport
  Last Stage : Inport  Port=2
  Bias : Bias  Bias=1
  Bias1 : Bias  Bias=+1
  Gain : Gain  Gain=-1
  Gain1 : Gain  Gain=-1
  Isp11 : Constant
  Isp15 : Constant  Value=0
  Isp16 : Constant  Value=Throttle
  Isp9 : Constant  Value=Throttle
  Product2 : Product
  Relational Operator1 : RelationalOperator  OutDataTypeStr=boolean
  Sum2 : Sum  Inputs=|++
  Switch3 : Switch  Criteria=u2 > Threshold
  Switch5 : Switch  Criteria=u2 > Threshold
  Throttle_Scope : Scope
      settings: SaveName=ScopeData2
  Throttle : Outport
  wires:
  Relational Operator1/1 -> Switch3/2
  Isp11/1 -> Switch3/1
  [TOR] -> Switch5/2
  Switch3/1 -> Switch5/3
  Switch5/1 -> Throttle/1, Throttle_Scope/1
  Isp15/1 -> Switch5/1
  Isp16/1 -> Gain/1
  Gain/1 -> Bias/1
  Bias/1 -> Product2/1
  Bias1/1 -> Product2/2
  Isp9/1 -> Sum2/1
  Product2/1 -> Sum2/2
  Sum2/1 -> Switch3/3
  [Qper] -> Gain1/1
  Gain1/1 -> Bias1/1
  Current Stage/1 -> Relational Operator1/1
  Last Stage/1 -> Relational Operator1/2

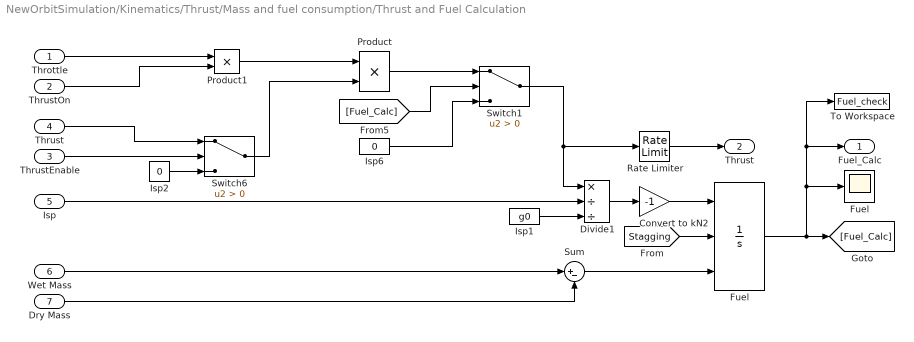
== system NewOrbitSimulation/Kinematics/Thrust/Mass and fuel consumption/Thrust and Fuel Calculation ==
  Throttle : Inport
  ThrustOn : Inport  Port=2
  ThrustEnable : Inport  Port=3
  Thrust : Inport  Port=4
  Isp : Inport  Port=5
  Wet Mass : Inport  Port=6
  Dry Mass : Inport  Port=7
  Convert to kN2 : Gain  Gain=-1
  Divide1 : Product  Inputs=*//
  Fuel : Integrator  ExternalReset=rising  InitialConditionSource=external  LimitOutput=on  LowerSaturationLimit=0
  "Fuel " : Scope
      settings: SaveName=ScopeData4
  Isp1 : Constant  Value=g0
  Isp2 : Constant  Value=0
  Isp6 : Constant  Value=0
  Product : Product
  Product1 : Product
  Rate Limiter : RateLimiter  RisingSlewLimit=100000  FallingSlewLimit=-100000  SampleTimeMode=inherited
  Sum : Sum  Inputs=|+-
  Switch1 : Switch  Criteria=u2 > Threshold
  Switch6 : Switch  Criteria=u2 > Threshold
  To Workspace : ToWorkspace  VariableName=Fuel_check  SampleTime=-1
      settings: MaxDataPoints=1
  Fuel_Calc : Outport
  "Thrust " : Outport  Port=2
  wires:
  Isp1/1 -> Divide1/3
  Divide1/1 -> Convert to kN2/1
  Convert to kN2/1 -> Fuel/1
  Sum/1 -> Fuel/3
  Wet Mass/1 -> Sum/1
  Dry Mass/1 -> Sum/2
  Switch6/1 -> Product/2
  [Stagging] -> Fuel/2
  Switch1/1 -> Rate Limiter/1, Divide1/1
  Product/1 -> Switch1/1
  ThrustOn/1 -> Product1/2
  Product1/1 -> Product/1
  Rate Limiter/1 -> "Thrust "/1
  [Fuel_Calc] -> Switch1/2
  Isp6/1 -> Switch1/3
  Throttle/1 -> Product1/1
  Fuel/1 -> [Fuel_Calc], "Fuel "/1, To Workspace/1, Fuel_Calc/1
  ThrustEnable/1 -> Switch6/2
  Isp/1 -> Divide1/2
  Isp2/1 -> Switch6/3
  Thrust/1 -> Switch6/1

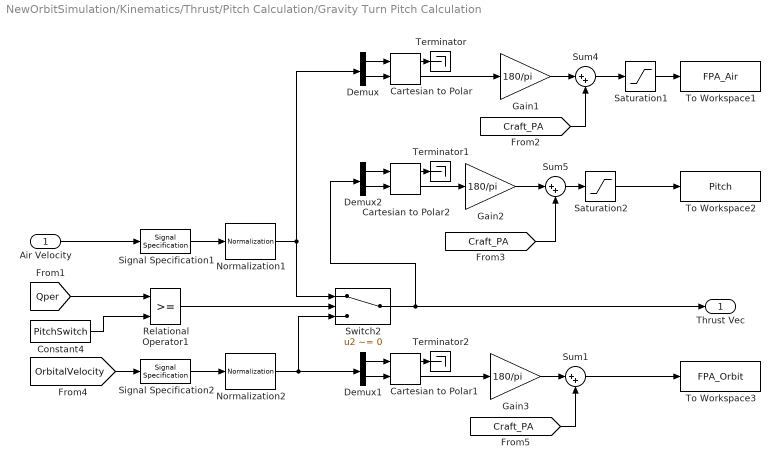
== system NewOrbitSimulation/Kinematics/Thrust/Pitch Calculation/Gravity Turn Pitch Calculation ==
  Air Velocity : Inport
  Cartesian to Polar : simulink_extras/Transformations/Cartesian to Polar
  Cartesian to Polar1 : simulink_extras/Transformations/Cartesian to Polar
  Cartesian to Polar2 : simulink_extras/Transformations/Cartesian to Polar
  Constant4 : Constant  Value=PitchSwitch
  Demux : Demux  Outputs=2
  Demux1 : Demux  Outputs=2
  Demux2 : Demux  Outputs=2
  Gain1 : Gain  Gain=180/pi
  Gain2 : Gain  Gain=180/pi
  Gain3 : Gain  Gain=180/pi
  Normalization1 : dspmathops/Normalization  NormType=2-norm  Bias=1e-10  NormOver=Specified dimension  ColComp=off  Dimension=1  outputMin=[]  outputMax=[]  accumDataTypeStr=Inherit: Same as product output  accumLastDataTypeStr=Inherit: Same as product output  roundingMode=Floor  overflowMode=off
  Normalization2 : dspmathops/Normalization  NormType=2-norm  Bias=1e-10  NormOver=Specified dimension  ColComp=off  Dimension=1  outputMin=[]  outputMax=[]  accumDataTypeStr=Inherit: Same as product output  accumLastDataTypeStr=Inherit: Same as product output  roundingMode=Floor  overflowMode=off
  Relational Operator1 : RelationalOperator  OutDataTypeStr=boolean
  Saturation1 : Saturate  UpperLimit=90  LowerLimit=0
  Saturation2 : Saturate  UpperLimit=90  LowerLimit=0
  Signal Specification1 : SignalSpecification  Dimensions=2
  Signal Specification2 : SignalSpecification  Dimensions=2
  Sum1 : Sum  Inputs=|++
  Sum4 : Sum  Inputs=|++
  Sum5 : Sum  Inputs=|++
  Switch2 : Switch  Criteria=u2 ~= 0  Threshold=PitchOverAlt
  Terminator : Terminator
  Terminator1 : Terminator
  Terminator2 : Terminator
  To Workspace1 : ToWorkspace  VariableName=FPA_Air  SampleTime=-1
  To Workspace2 : ToWorkspace  VariableName=Pitch  SampleTime=-1
  To Workspace3 : ToWorkspace  VariableName=FPA_Orbit  SampleTime=-1
  Thrust Vec : Outport
  wires:
  [Qper] -> Relational Operator1/1
  Relational Operator1/1 -> Switch2/2
  Normalization1/1 -> Switch2/1, Demux/1
  Demux1/1 -> Cartesian to Polar1/1
  Switch2/1 -> Thrust Vec/1, Demux2/1
  Constant4/1 -> Relational Operator1/2
  Cartesian to Polar/1 -> Terminator/1
  Sum1/1 -> To Workspace3/1
  Air Velocity/1 -> Signal Specification1/1
  Demux/2 -> Cartesian to Polar/2
  Signal Specification2/1 -> Normalization2/1
  Normalization2/1 -> Demux1/1, Switch2/3
  Signal Specification1/1 -> Normalization1/1
  Demux/1 -> Cartesian to Polar/1
  Demux1/2 -> Cartesian to Polar1/2
  Cartesian to Polar1/1 -> Terminator2/1
  [OrbitalVelocity] -> Signal Specification2/1
  Gain1/1 -> Sum4/1
  Cartesian to Polar1/2 -> Gain3/1
  Gain3/1 -> Sum1/1
  [Craft_PA] -> Sum1/2
  Saturation2/1 -> To Workspace2/1
  Cartesian to Polar/2 -> Gain1/1
  Cartesian to Polar2/1 -> Terminator1/1
  Saturation1/1 -> To Workspace1/1
  Gain2/1 -> Sum5/1
  [Craft_PA] -> Sum5/2
  Sum5/1 -> Saturation2/1
  Demux2/1 -> Cartesian to Polar2/1
  Cartesian to Polar2/2 -> Gain2/1
  Demux2/2 -> Cartesian to Polar2/2
  [Craft_PA] -> Sum4/2
  Sum4/1 -> Saturation1/1

== system NewOrbitSimulation/Kinematics/Thrust/Pitch Calculation/Subsystem ==
  Position : Inport
  Altitude : Inport  Port=2
  Gain : Gain  Gain=-pi/180
  Linear Pitch Over : Gain  Gain=PitchOverAngle/PitchOverAlt
  Normalization : dspmathops/Normalization  NormType=2-norm  Bias=1e-10  NormOver=Specified dimension  ColComp=off  Dimension=1  outputMin=[]  outputMax=[]  accumDataTypeStr=Inherit: Same as product output  accumLastDataTypeStr=Inherit: Same as product output  roundingMode=Floor  overflowMode=off
  Saturation : Saturate  UpperLimit=90  LowerLimit=0
  Signal Specification : SignalSpecification  Dimensions=2
  Vector Rotation 2D : Subsystem
  Up Vector : Outport
  wires:
  Altitude/1 -> Linear Pitch Over/1
  Position/1 -> Signal Specification/1
  Signal Specification/1 -> Normalization/1
  Normalization/1 -> Vector Rotation 2D/1(Position)
  Saturation/1 -> Gain/1
  Gain/1 -> Vector Rotation 2D/2(Phase Angle)
  Linear Pitch Over/1 -> Saturation/1
  Vector Rotation 2D/1("Rotated Vector ") -> Up Vector/1

== system NewOrbitSimulation/Kinematics/Aerodynamics/Aerodynamic Calculations/Cl and Cd Calculation/Air Velocity Vector Normalized ==
  Vector : Inport
  Constant : Constant
  Demux3 : Demux  Outputs=2
  Divide1 : Product  Inputs=*/
  Divide2 : Product  Inputs=*/
  Magnitude Calc : Subsystem
  Mux1 : Mux  Inputs=2
  Switch : Switch  Criteria=u2 > Threshold
  "Normalized " : Outport
  wires:
  Demux3/1 -> Divide1/1
  Vector/1 -> Demux3/1, Magnitude Calc/1(Vector)
  Mux1/1 -> "Normalized "/1
  Demux3/2 -> Divide2/1
  Constant/1 -> Switch/3
  Magnitude Calc/1("Magnitude ") -> Switch/1
  Magnitude Calc/2(Is Zero) -> Switch/2
  Divide1/1 -> Mux1/1
  Divide2/1 -> Mux1/2
  Switch/1 -> Divide2/2, Divide1/2

== system NewOrbitSimulation/Kinematics/Aerodynamics/Aerodynamic Calculations/Cl and Cd Calculation/Magnitude Calc ==
  Vector : Inport
  Add : Sum
  Demux : Demux  Outputs=2
  Math Function : Math  Operator=square  SaturateOnIntegerOverflow=on
  Math Function1 : Math  Operator=square  SaturateOnIntegerOverflow=on
  Sqrt : Sqrt  SaturateOnIntegerOverflow=on
  "Magnitude " : Outport
  wires:
  Demux/1 -> Math Function1/1
  Demux/2 -> Math Function/1
  Math Function/1 -> Add/2
  Add/1 -> Sqrt/1
  Vector/1 -> Demux/1
  Math Function1/1 -> Add/1
  Sqrt/1 -> "Magnitude "/1

== system NewOrbitSimulation/Kinematics/Aerodynamics/Aerodynamic Calculations/Cl and Cd Calculation/Magnitude Calc5 ==
  Vector : Inport
  Phase Angle : Inport  Port=2
  Add : Sum  Inputs=+-
  Add1 : Sum
  Demux : Demux  Outputs=2
  Mux : Mux  Inputs=2
  Product{,1..3} (4 alike) : Product
  Trigonometric Function : Trigonometry
  Trigonometric Function1 : Trigonometry  Operator=cos
  "Rotated Vector " : Outport
  wires:
  Mux/1 -> "Rotated Vector "/1
  Phase Angle/1 -> Trigonometric Function/1, Trigonometric Function1/1
  Vector/1 -> Demux/1
  Trigonometric Function1/1 -> Product3/2, Product/2
  Demux/1 -> Product2/2, Product/1
  Product/1 -> Add/1
  Demux/2 -> Product3/1, Product1/1
  Trigonometric Function/1 -> Product2/1, Product1/2
  Product1/1 -> Add/2
  Product2/1 -> Add1/1
  Product3/1 -> Add1/2
  Add1/1 -> Mux/2
  Add/1 -> Mux/1

== system NewOrbitSimulation/Kinematics/Aerodynamics/Aerodynamic Calculations/Magnitude Calc1/Magnitude Calc ==
  Vector : Inport
  Add : Sum
  Demux : Demux  Outputs=2
  Math Function : Math  Operator=square  SaturateOnIntegerOverflow=on
  Math Function1 : Math  Operator=square  SaturateOnIntegerOverflow=on
  Sqrt : Sqrt  SaturateOnIntegerOverflow=on
  "Magnitude " : Outport
  wires:
  Demux/1 -> Math Function1/1
  Demux/2 -> Math Function/1
  Math Function/1 -> Add/2
  Add/1 -> Sqrt/1
  Vector/1 -> Demux/1
  Math Function1/1 -> Add/1
  Sqrt/1 -> "Magnitude "/1

== system NewOrbitSimulation/Kinematics/Thrust/Pitch Calculation/Subsystem/Vector Rotation 2D ==
  Position : Inport
  Phase Angle : Inport  Port=2
  Add : Sum  Inputs=+-
  Add1 : Sum
  Demux : Demux  Outputs=2
  Mux : Mux  Inputs=2
  Product{,1..3} (4 alike) : Product
  Trigonometric Function : Trigonometry
  Trigonometric Function1 : Trigonometry  Operator=cos
  "Rotated Vector " : Outport
  wires:
  Mux/1 -> "Rotated Vector "/1
  Phase Angle/1 -> Trigonometric Function/1, Trigonometric Function1/1
  Position/1 -> Demux/1
  Trigonometric Function1/1 -> Product3/2, Product/2
  Demux/1 -> Product2/2, Product/1
  Product/1 -> Add/1
  Demux/2 -> Product3/1, Product1/1
  Trigonometric Function/1 -> Product2/1, Product1/2
  Product1/1 -> Add/2
  Product2/1 -> Add1/1
  Product3/1 -> Add1/2
  Add1/1 -> Mux/2
  Add/1 -> Mux/1

== system NewOrbitSimulation/Kinematics/Aerodynamics/Aerodynamic Calculations/Cl and Cd Calculation/Air Velocity Vector Normalized/Magnitude Calc ==
  Vector : Inport
  Add : Sum
  Constant : Constant
  Constant1 : Constant  Value=0
  Demux : Demux  Outputs=2
  Math Function : Math  Operator=square  SaturateOnIntegerOverflow=on
  Math Function1 : Math  Operator=square  SaturateOnIntegerOverflow=on
  Sqrt : Sqrt  SaturateOnIntegerOverflow=on
  Switch : Switch  Criteria=u2 ~= 0
  "Magnitude " : Outport
  Is Zero : Outport  Port=2
  wires:
  Demux/1 -> Math Function1/1
  Demux/2 -> Math Function/1
  Math Function/1 -> Add/2
  Add/1 -> Sqrt/1
  Vector/1 -> Demux/1
  Math Function1/1 -> Add/1
  Switch/1 -> Is Zero/1
  Constant/1 -> Switch/1
  Constant1/1 -> Switch/3
  Sqrt/1 -> Switch/2, "Magnitude "/1

== matlab function NewOrbitSimulation/Orbital Mechanics Calculations/Orbital Mechanics ==
  data: h output; eta_to_ap output; a output; OrbitalSpeed input; Vvert input; ecc output size=1; Altitude input; GM_planet parameter size=1; Ra output size=1; Rp output size=1; R_planet parameter; GndAlt_planet parameter
function [h,eta_to_ap,a,ecc,Ra,Rp] = fcn(OrbitalSpeed,Vvert,Altitude,GM_planet,R_planet,GndAlt_planet)
%#codegen
Radius = Altitude + R_planet;
Vpar = Vvert;
Vper = sqrt(abs(OrbitalSpeed^2 - Vpar^2));
h = Radius*Vper;

E = OrbitalSpeed^2/2 - GM_planet/Radius;
a = -GM_planet/(2*E);

ecc = sqrt(abs(1-((-2*E)*h^2)/(GM_planet^2)));

Ra = a*(1 + ecc) - (R_planet - GndAlt_planet);
Rp = a*(1 - ecc) - (R_planet - GndAlt_planet);

Theta = acosd(complex((1/ecc)*((h^2)/(GM_planet*Radius) - 1)));
%Theta = 0;
n = sqrt(abs(GM_planet/(a^3)));

EA = 2*atand(sqrt(abs(((1-ecc)/(1+ecc))*(tand(Theta/2)))));

MA = EA*pi/180 - ecc*sind(EA);
Delta_MA = pi - MA;

eta_to_ap = Delta_MA/n;

== stateflow chart NewOrbitSimulation/Kinematics/Thrust/Mass and fuel consumption/Chart ==
  settings: executeAtInitialization=1  initializeOutput=1
  state Start
    entry: Stage = 1;
  state Stage_Rocket_finish
    entry: ThrustToggle = 0
    entry: Stagging = 0
  state Nominal
    entry: ThrustToggle = 1;
    entry: Stagging = 0;
    entry: CurrentStage = Stage;
    entry: WetMass = ThrustMassData(Stage,1);
    entry: DryMass = ThrustMassData(Stage,2);
    entry: Thrust = ThrustMassData(Stage,3);
    entry: Isp = ThrustMassData(Stage,4);
  state Stage_Rocket
    entry: ThrustToggle = 0;
    entry: Stagging = 1;
    entry: Stage = Stage + 1;
    entry: WetMass = ThrustMassData(Stage,1);
    entry: DryMass = ThrustMassData(Stage,2);
    entry: Thrust = ThrustMassData(Stage,3);
    entry: Isp = ThrustMassData(Stage,4);
  (default) -> Start
  Start -> Nominal : [Stage == 1]
  Nominal -> Stage_Rocket_finish [order 2] : [OutOfFuel == 1 && Stage == LastStage]
  Nominal -> Stage_Rocket [order 1] : [OutOfFuel == 1 && Stage < LastStage]
  Stage_Rocket -> Nominal : [OutOfFuel == 0 && Stage <= LastStage]
  data: OutOfFuel input; ThrustToggle output; Stagging output; LastStage input; Stage local; WetMass output; DryMass output; Thrust output; Isp output; ThrustMassData parameter; CurrentStage output
